simulink model "PowerWindow_v5"  (R2021a)
settings: Solver=VariableStepAuto  StartTime=0.0  StopTime=20  RelTol=1e-3
model workspace (MAT data in the model file):
  B = 0.01
  Ke_phi = 1.6
  Ra = 0.5
  TL = 20
  tau_a1 = 0.2
  tau_m = 500
settings Model: EnablePacing=on  PacingRate=0.630000  Creator=achu  LastModifiedBy=achu

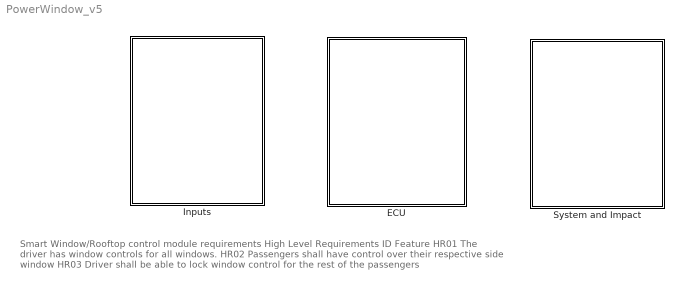
== system PowerWindow_v5 ==
  note: Smart Window/Rooftop control module requirements
      |
      | High Level Requirements
      |
      | ID
      | Feature
      |
      | HR01
      | The driver has window controls for all windows.
      |
      | HR02
      | Passengers shall have control over their respective side window
      |
      | HR03
      | Driver shall be able to lock window control for the rest of the passengers
  ECU : Subsystem
  Inputs : Subsystem
  System and Impact : Subsystem

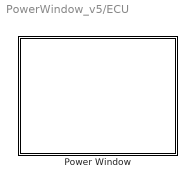
== system PowerWindow_v5/ECU ==
  Power Window : Subsystem  ReferencedSubsystem=Power_Window_ECU

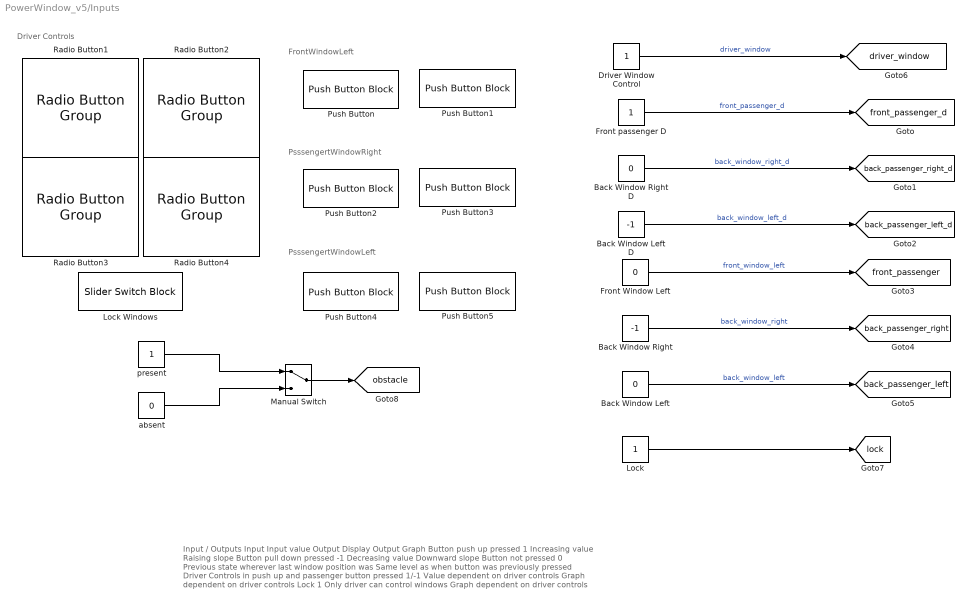
== system PowerWindow_v5/Inputs ==
  note: Input / Outputs
      |
      | Input
      | Input value
      | Output Display
      | Output Graph
      |
      | Button push up pressed
      | 1
      | Increasing value
      | Raising slope
      |
      | Button pull down pressed
      | -1
      | Decreasing value
      | Downward slope
      |
      | Button not pressed
      | 0
      | Previous state wherever last window position was
      | Same level as when button was previously pressed
      |
      | Driver Controls in push up and passenger button pressed
      | 1/-1
      | Value dependent on driver controls
      | Graph dependent on driver controls
      |
      | Lock
      | 1
      | Only driver can control windows
      | Graph dependent on driver controls
  note: FrontWindowLeft
  note: Driver Controls
  note: PsssengertWindowRight
  note: PsssengertWindowLeft
  Back Window Left : Constant  Value=0
  Back Window Left D : Constant  Value=-1
  Back Window Right : Constant  Value=-1
  Back Window Right D : Constant  Value=0
  Driver Window Control : Constant
  Front Window Left : Constant  Value=0
  Front passenger D : Constant
  Lock : Constant
  Lock Windows : SliderSwitchBlock
      settings: Values={{'Unlock', 'Lock'}, [0 1]}
  Manual Switch : ManualSwitch
  Push Button : PushButtonBlock  ButtonText=Push up window
  Push Button1 : PushButtonBlock  ButtonText=Pull down window  OnValue=-1
  Push Button2 : PushButtonBlock  ButtonText=Push up window
  Push Button3 : PushButtonBlock  ButtonText=Pull down window  OnValue=-1
  Push Button4 : PushButtonBlock  ButtonText=Push up window
  Push Button5 : PushButtonBlock  ButtonText=Pull down window  OnValue=-1
  Radio Button1 : RadioButtonGroup  LabelPosition=Hide  SelectedLabel=Open  ButtonGroupName=Driver Window Controls
      settings: Values={{'Open', 'Stop', 'Close'}, [1 0 -1]}
  Radio Button2 : RadioButtonGroup  LabelPosition=Hide  SelectedLabel=Open  ButtonGroupName=Front Passenger
      settings: Values={{'Open', 'Stop', 'Close'}, [1 0 -1]}
  Radio Button3 : RadioButtonGroup  LabelPosition=Hide  SelectedLabel=Stop  ButtonGroupName=Back Window Right
      settings: Values={{'Open', 'Stop', 'Close'}, [1 0 -1]}
  Radio Button4 : RadioButtonGroup  LabelPosition=Hide  SelectedLabel=Close  ButtonGroupName=Back Window Left
      settings: Values={{'Open', 'Stop', 'Close'}, [1 0 -1]}
  absent : Constant  Value=0
  present : Constant
  tag scope: back_passenger_left=global, back_passenger_left_d=global, back_passenger_right=global, back_passenger_right_d=global, driver_window=global, front_passenger=global, front_passenger_d=global, lock=global, obstacle=global
  wires:
  Front passenger D/1 -> [front_passenger_d]  "front_passenger_d"
  Back Window Left/1 -> [back_passenger_left]  "back_window_left"
  Back Window Right/1 -> [back_passenger_right]  "back_window_right"
  Lock/1 -> [lock]
  Back Window Left D/1 -> [back_passenger_left_d]  "back_window_left_d"
  present/1 -> Manual Switch/1
  Back Window Right D/1 -> [back_passenger_right_d]  "back_window_right_d"
  Manual Switch/1 -> [obstacle]
  Front Window Left/1 -> [front_passenger]  "front_window_left"
  Driver Window Control/1 -> [driver_window]  "driver_window"
  absent/1 -> Manual Switch/2

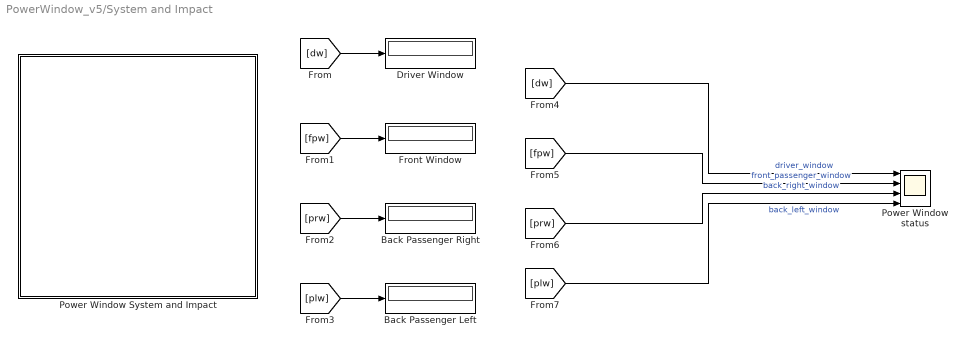
== system PowerWindow_v5/System and Impact ==
  Back Passenger Left : Display
  Back Passenger Right : Display
  Driver Window : Display
  Front Window : Display
  Power Window System and Impact : Subsystem  ReferencedSubsystem=Power_Window_System_and_Impact
  Power Window status : Scope  NumInputPorts=4
  wires:
  [dw] -> Driver Window/1
  [fpw] -> Front Window/1
  [prw] -> Back Passenger Right/1
  [plw] -> Back Passenger Left/1
  [fpw] -> Power Window status/2  "front_passenger_window"
  [prw] -> Power Window status/3  "back_right_window"
  [dw] -> Power Window status/1  "driver_window"
  [plw] -> Power Window status/4  "back_left_window"
